simulink model "ForceControl"  (R2018a)
settings: Solver=VariableStepAuto  StartTime=0.0  StopTime=inf  RelTol=1e-3
undefined symbols (not defined in the file): X, Y, Z
libraries: robotlib x7
settings Model: Creator=ryodo  LastModifiedBy=ryodo

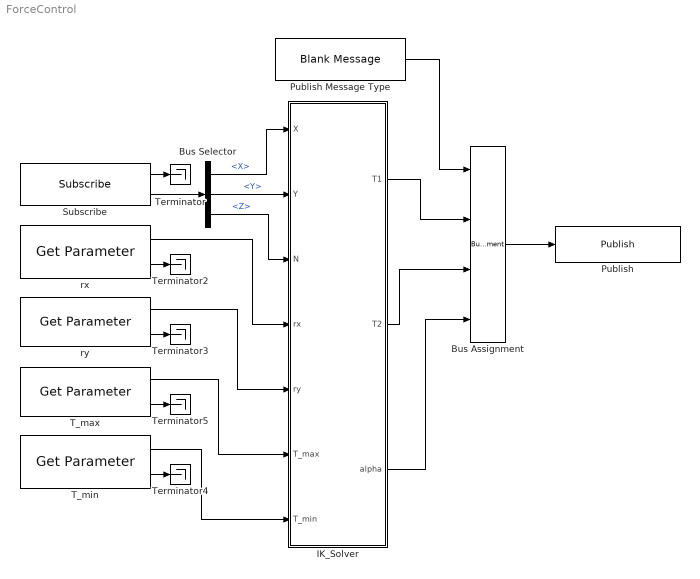
== system ForceControl ==
  Bus Assignment : BusAssignment  AssignedSignals=X,Y,Z
  Bus Selector : BusSelector  OutputSignals=X,Y,Z
  IK_Solver : MATLAB Function  TreatAsAtomicUnit=on
  Publish : robotlib/Publish  SourceLibraryInfo=This block requires Robotics System Toolbox  topicSource=Specify your own  topic=/result_force  messageType=geometry_msgs/Vector3  messageQueueLength=1
      settings: SourceProductBaseCode=RO
  Publish Message Type : robotlib/Blank Message  SourceLibraryInfo=This block requires Robotics System Toolbox  messageType=geometry_msgs/Vector3  SampleTime=-1
      settings: SourceProductBaseCode=RO
  Subscribe : robotlib/Subscribe  SourceLibraryInfo=This block requires Robotics System Toolbox  topicSource=Specify your own  topic=/cmd_force  messageType=geometry_msgs/Vector3  sampleTime=-1  messageQueueLength=1
      settings: SourceProductBaseCode=RO
  T_max : robotlib/Get Parameter  SourceLibraryInfo=This block requires Robotics System Toolbox  ParameterSource=Specify your own  ParameterName=/wam_v/T_max  ParameterType=double  ParameterMaxArrayLength=16  ParameterInitialValue=0.0  SampleTime=-1  ShowErrorCodeOutput=on  ModelName=ForceControl  BlockId=ParamGet_ForceControl_20
      settings: SourceProductName=Robotics System Toolbox  SourceProductBaseCode=RO
  T_min : robotlib/Get Parameter  SourceLibraryInfo=This block requires Robotics System Toolbox  ParameterSource=Specify your own  ParameterName=/wam_v/T_min  ParameterType=double  ParameterMaxArrayLength=16  ParameterInitialValue=0.0  SampleTime=-1  ShowErrorCodeOutput=on  ModelName=ForceControl  BlockId=ParamGet_ForceControl_21
      settings: SourceProductName=Robotics System Toolbox  SourceProductBaseCode=RO
  Terminator{,2..5} (5 alike) : Terminator
  rx : robotlib/Get Parameter  SourceLibraryInfo=This block requires Robotics System Toolbox  ParameterSource=Specify your own  ParameterName=/wam_v/rx  ParameterType=double  ParameterMaxArrayLength=16  ParameterInitialValue=0.0  SampleTime=-1  ShowErrorCodeOutput=on  ModelName=ForceControl  BlockId=ParamGet_ForceControl_18
      settings: SourceProductName=Robotics System Toolbox  SourceProductBaseCode=RO
  "ry " : robotlib/Get Parameter  SourceLibraryInfo=This block requires Robotics System Toolbox  ParameterSource=Specify your own  ParameterName=/wam_v/ry  ParameterType=double  ParameterMaxArrayLength=16  ParameterInitialValue=0.0  SampleTime=-1  ShowErrorCodeOutput=on  ModelName=ForceControl  BlockId=ParamGet_ForceControl_19
      settings: SourceProductName=Robotics System Toolbox  SourceProductBaseCode=RO
  wires:
  Subscribe/2 -> Bus Selector/1
  Bus Selector/1 -> IK_Solver/1(X)  "<X>"
  Bus Selector/2 -> IK_Solver/2(Y)  "<Y>"
  Bus Selector/3 -> IK_Solver/3(N)  "<Z>"
  Subscribe/1 -> Terminator/1
  IK_Solver/2(T2) -> Bus Assignment/3
  IK_Solver/3(alpha) -> Bus Assignment/4
  Bus Assignment/1 -> Publish/1
  Publish Message Type/1 -> Bus Assignment/1
  IK_Solver/1(T1) -> Bus Assignment/2
  rx/2 -> Terminator2/1
  "ry "/2 -> Terminator3/1
  T_min/2 -> Terminator4/1
  T_max/2 -> Terminator5/1
  rx/1 -> IK_Solver/4(rx)
  "ry "/1 -> IK_Solver/5(ry)
  T_max/1 -> IK_Solver/6(T_max)
  T_min/1 -> IK_Solver/7(T_min)

== matlab function ForceControl/IK_Solver ==
  data: X input double size=1; T1 output double size=1; Y input double size=1; N input double size=1; T2 output double size=1; alpha output double size=1; rx input; ry input; T_max input; T_min input
function [ T1, T2, alpha ] = IK_Solver(X, Y, N, rx, ry, T_max, T_min)
    int8 x;
    int8 y;
    int8 n;
    x = 1 * int8(not(X==0));
    y = 2 * int8(not(Y==0));
    n = 4 * int8(not(N==0));

    switch x+y+n
        case 0
            T1=0;
            T2=0;
            alpha=0;
        case 1
            T1=X/2;
            T2=T1;
            alpha=0;
        case 2
            T1=Y/sqrt(2);
            T2=-T1;
            alpha=pi/4;
        case 3
            T1=(X+Y)/sqrt(2);
            T2=(X-Y)/sqrt(2);
            alpha=pi/4;
        case 4
            T1=N/(2*rx);
            T2=-T1;
            alpha=0;
        case 5
            T1=(X+(N/rx))/2;
            T2=(X-(N/rx))/2;
            alpha=0;
        case 6
            alpha=abs(atan((rx*Y)/(N+ry*Y)));
            double Ttmp_Y;
            double Ttmp_N;
            Ttmp_Y=Y/(2*sin(alpha));
            Ttmp_N=N/( 2*( rx*cos(alpha)-ry*sin(alpha) ) );
            if( (Ttmp_Y <= T_min || T_max <= Ttmp_Y) && (Ttmp_N <= T_min || T_max <= Ttmp_N) )
                T1=0;
                T2=0;
                alpha=0;
            elseif (Ttmp_Y <= T_min || T_max <= Ttmp_Y)
                T1=N/(2*rx);
                T2=-T1;
                alpha=0;
            elseif (Ttmp_N <= T_min || T_max <= Ttmp_N)
                T1=Y/sqrt(2);
                T2=-T1;
                alpha=pi/4;
            else
                T1=Ttmp_Y;
                T2=-T1;
            end
        case 7
            alpha=abs(atan((rx*Y)/(N+ry*Y)));
            double T1_tmp_Y;
            double T1_tmp_N;
            double T2_tmp_Y;
            double T2_tmp_N;
            T1_tmp_Y=X/(2*cos(alpha)) + Y/(2*sin(alpha));
            T1_tmp_N=X/(2*cos(alpha)) + N/( 2*(rx*cos(alpha)-ry*sin(alpha) ) );
            T2_tmp_Y=X/(2*cos(alpha)) - Y/(2*sin(alpha));    
            T2_tmp_N=X/(2*cos(alpha)) - N/( 2*(rx*cos(alpha)-ry*sin(alpha) ) );

            if( ( (T1_tmp_Y <= T_min || T_max <= T1_tmp_Y) || (T2_tmp_Y <= T_min || T_max <= T2_tmp_Y) ) && ( (T1_tmp_N <= T_min || T_max <= T1_tmp_N) || (T2_tmp_N <= T_min || T_max <= T2_tmp_N) ) )
                T1=0;
                T2=0;
                alpha=0;
            elseif ( (T1_tmp_Y <= T_min || T_max <= T1_tmp_Y) || (T2_tmp_Y <= T_min || T_max <= T2_tmp_Y) )
                T1=(X+(N/rx))/2;
                T2=(X-(N/rx))/2;
                alpha=0;
            elseif ( (T1_tmp_N <= T_min || T_max <= T1_tmp_N) || (T2_tmp_N <= T_min || T_max <= T2_tmp_N) )
                T1=(X+Y)/sqrt(2);
                T2=(X-Y)/sqrt(2);
                alpha=pi/4;
            else
                T1=T1_tmp_Y;
                T2=T2_tmp_Y;
            end
        otherwise
            T1=0;
            T2=0;
            alpha=0;
    end
    
%     Limit 
    if (T1 <= T_min)
        T1=T_min;
    end
    if (T_max <= T1)
        T1=T_max;
    end
    if (T2 <= T_min)
        T2=T_min;
    end
    if (T_max <= T2)
        T2=T_max;
    end
    if (alpha <= 0)
        alpha=0;
    end
    if (pi/2 <= alpha)
       alpha=pi/2;
    end
